simulink model "EXAMPLE"  (R2018b)
settings: Solver=ode4  StartTime=0.0  StopTime=1.8  FixedStep=50e-6  RelTol=1e-3
libraries: simulink x5, powerlib_meascontrol x5, dsparch4 x4
settings Model: Creator=Пользователь  LastModifiedBy=Пользователь

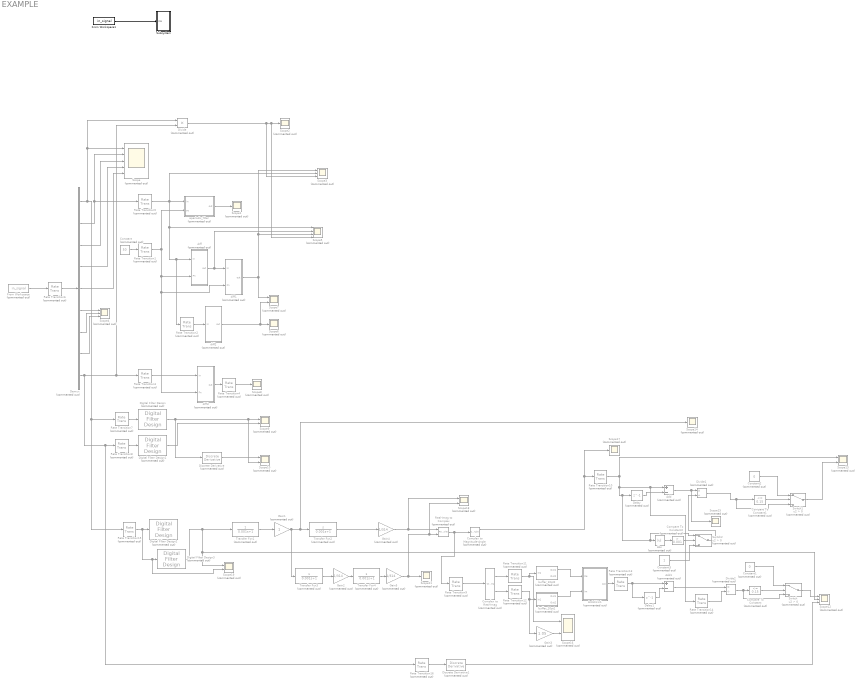
== system EXAMPLE ==
  Abs : Abs  Commented=on
  Add : Sum  Commented=on  Inputs=+-
  Add1 : Sum  Commented=on  Inputs=+-
  Antishkin1 : MATLAB Function  Commented=on  TreatAsAtomicUnit=on
  Compare To Constant : simulink/Logic and Bit Operations/Compare To Constant  Commented=on  relop=<=  const=0.15  OutDataTypeStr=boolean
  Compare To Constant1 : simulink/Logic and Bit Operations/Compare To Constant  Commented=on  relop=<=  const=0.15  OutDataTypeStr=boolean
  Compare To Constant2 : simulink/Logic and Bit Operations/Compare To Constant  Commented=on  relop=>  const=0.001  OutDataTypeStr=boolean
  Complex to Magnitude-Angle : ComplexToMagnitudeAngle  Commented=on
  Complex to Real-Imag : ComplexToRealImag  Commented=on
  Constant : Constant  Commented=on  Value=50
  Constant1 : Constant  Commented=on  Value=0
  Constant2 : Constant  Commented=on  Value=0
  Constant3 : Constant  Commented=on
  Delay : Delay  Commented=on  DelayLength=1
  Delay1 : Delay  Commented=on  DelayLength=1
  Demux : Demux  Commented=on  Outputs=9
  Digital Filter Design{,1..3} (4 alike) : dsparch4/Digital Filter Design  Commented=on  mwdsp_browser_bugfix_var=off
  Discrete Derivative : simulink/Discrete/Discrete Derivative  Commented=on  gainval=1.0  ICPrevScaledInput=0.0  OutMin=[]  OutMax=[]  OutDataType=fixdt(1, 16)  OutScaling=2^-10  DoSatur=off
  Discrete Derivative1 : simulink/Discrete/Discrete Derivative  Commented=on  gainval=1.0  ICPrevScaledInput=0.0  OutMin=[]  OutMax=[]  OutDataType=fixdt(1, 16)  OutScaling=2^-10  DoSatur=off
  Divide : Product  Commented=on  Inputs=**
  Divide1 : Product  Commented=on  Inputs=*/
  Divide2 : Product  Commented=on  Inputs=*/
  From Workspace : FromWorkspace  Commented=on  VariableName=in_signal  OutDataTypeStr=double  SampleTime=1/10000  OutputAfterFinalValue=Setting to zero
  From Workspace1 : FromWorkspace  VariableName=in_signal  OutDataTypeStr=double  SampleTime=1/10000  OutputAfterFinalValue=Setting to zero
  Gain1 : Gain  Commented=on
  Gain2 : Gain  Commented=on  Gain=1/314
  Gain3 : Gain  Commented=on  Gain=1.05
  Gain4 : Gain  Commented=on  Gain=1/314
  Gain5 : Gain  Commented=on  Gain=1/314
  Rate Transition{1..5,7..16} (15 alike) : RateTransition  Commented=on  OutPortSampleTime=1/4000
  Rate Transition6 : RateTransition  Commented=on  OutPortSampleTime=1/20000
  Real-Imag to Complex : RealImagToComplex  Commented=on
  Scope : Scope  Commented=on  NumInputPorts=5
  Scope{1..2,6,8,11,14..15,17} (8 alike) : Scope  Commented=on
  Scope{7,9..10,13,16,18..19} (7 alike) : Scope  Commented=on  NumInputPorts=2
  Scope12 : Scope  Commented=on  NumInputPorts=3
  Scope3 : Scope  Commented=on  NumInputPorts=3
  Scope4 : Scope  Commented=on  NumInputPorts=3
  Scope5 : Scope  Commented=on  NumInputPorts=4
  Subsystem : Subsystem
  Switch : Switch  Commented=on  Criteria=u2 > Threshold
  Switch1 : Switch  Commented=on  Criteria=u2 > Threshold
  Switch2 : Switch  Commented=on  Criteria=u2 > Threshold
  Transfer Fcn1 : TransferFcn  Commented=on  Numerator=1  Denominator=[0.001 1]
  Transfer Fcn2 : TransferFcn  Commented=on  Numerator=[1 0]  Denominator=[0.001 1]
  Transfer Fcn3 : TransferFcn  Commented=on  Numerator=[1 0]  Denominator=[0.001 1]
  Transfer Fcn4 : TransferFcn  Commented=on  Numerator=[1 0]  Denominator=[0.001 1]
  aperiodic_filter : Subsystem  Commented=on
  buffer_10pt1 : Subsystem  Commented=on
  buffer_10pt2 : Subsystem  Commented=on
  diff : Subsystem  Commented=on
  diff1 : Subsystem  Commented=on
  diff2 : Subsystem  Commented=on
  diff3 : Subsystem  Commented=on
  wires:
  Demux/2 -> Rate Transition5/1, Scope/2
  Demux/3 -> Scope/3
  Demux/4 -> Scope/4
  Demux/5 -> Scope/5
  aperiodic_filter/1(out) -> Scope1/1
  Constant/1 -> Rate Transition1/1
  Rate Transition5/1 -> Rate Transition2/1, diff/1(in), Scope5/1, Scope3/2, aperiodic_filter/1(in)
  Rate Transition1/1 -> aperiodic_filter/2(Fn), diff1/2(Fn), diff3/2(Fn), diff/2(Fn)
  diff/1(out) -> Scope5/2, diff1/1(in)
  diff1/1(out) -> Scope3/1, Scope5/3, Scope7/1
  Divide/1 -> Scope3/3, Scope5/4, Scope2/1
  Demux/6 -> Scope4/1
  Demux/7 -> Scope4/2
  Demux/8 -> Scope4/3
  diff2/1(out) -> Scope7/2, Scope6/1
  Rate Transition2/1 -> diff2/1(in)
  diff3/1(out) -> Rate Transition4/1
  Rate Transition3/1 -> diff3/1(in)
  Rate Transition4/1 -> Scope8/1
  Rate Transition6/1 -> Demux/1
  From Workspace/1 -> Rate Transition6/1
  Rate Transition7/1 -> Digital Filter Design/1
  Rate Transition8/1 -> Digital Filter Design1/1
  Digital Filter Design/1 -> Discrete Derivative/1, Scope10/2, Scope9/1
  Digital Filter Design1/1 -> Scope9/2
  Discrete Derivative/1 -> Scope10/1
  Transfer Fcn1/1 -> Gain1/1
  Complex to Magnitude-Angle/1 -> Scope17/1, Rate Transition10/1
  Real-Imag to Complex/1 -> Rate Transition9/1, Complex to Magnitude-Angle/1
  Rate Transition10/1 -> Scope13/1, Rate Transition14/1, Add/1, Switch2/1, Abs/1, Delay/1
  Transfer Fcn3/1 -> Gain2/1
  Complex to Real-Imag/1 -> Rate Transition11/1
  Complex to Real-Imag/2 -> Rate Transition12/1
  buffer_10pt2/1(Out1) -> Antishkin1/1(Re)
  buffer_10pt1/1(Out1) -> Antishkin1/2(Im)
  Gain1/1 -> Transfer Fcn3/1, Transfer Fcn2/1, Scope14/1
  Gain3/1 -> Scope16/2
  Demux/1 -> Rate Transition15/1, Rate Transition7/1, Divide/1, Scope/1
  Rate Transition9/1 -> Complex to Real-Imag/1
  Delay/1 -> Add/2
  Add/1 -> Scope15/1, Divide1/1
  Antishkin1/1(out) -> Rate Transition13/1
  Divide2/1 -> Switch/3, Compare To Constant/1
  Rate Transition11/1 -> Scope16/1, buffer_10pt2/1(In1)
  Rate Transition12/1 -> Gain3/1, buffer_10pt1/1(In1)
  Add1/1 -> Divide2/1
  Rate Transition14/1 -> Divide2/2
  Demux/9 -> Rate Transition16/1, Rate Transition8/1, Divide/2, Rate Transition3/1
  Compare To Constant/1 -> Switch/2
  Constant1/1 -> Switch/1
  Switch/1 -> Scope12/1
  Constant2/1 -> Switch1/1
  Compare To Constant1/1 -> Switch1/2
  Divide1/1 -> Switch1/3, Compare To Constant1/1
  Switch1/1 -> Scope13/2
  Rate Transition13/1 -> Delay1/1, Add1/1
  Delay1/1 -> Add1/2
  Gain5/1 -> Scope11/1, Scope18/2, Real-Imag to Complex/2
  Digital Filter Design3/1 -> Scope19/1, Scope12/2, Transfer Fcn1/1
  Rate Transition15/1 -> Scope19/2, Digital Filter Design3/1, Digital Filter Design2/1
  Transfer Fcn2/1 -> Gain4/1
  Gain4/1 -> Scope18/1, Real-Imag to Complex/1
  Gain2/1 -> Transfer Fcn4/1
  Transfer Fcn4/1 -> Gain5/1
  Discrete Derivative1/1 -> Scope12/3
  Rate Transition16/1 -> Discrete Derivative1/1
  Compare To Constant2/1 -> Switch2/2
  Switch2/1 -> Divide1/2
  Abs/1 -> Compare To Constant2/1
  Constant3/1 -> Switch2/3
  From Workspace1/1 -> Subsystem/1(In1)

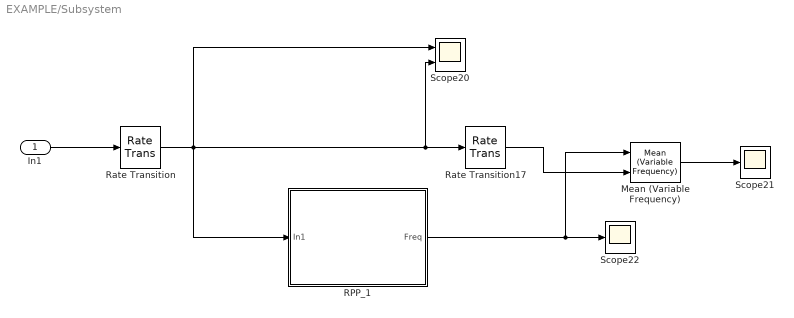
== system EXAMPLE/Subsystem ==
  In1 : Inport
  Mean (Variable Frequency) : powerlib_meascontrol/Measurements/Mean (Variable Frequency)  Finit=50  Fmin=45  Vinit=0  Ts=1/4000
      settings: SourceProductName=Simscape Power Systems  SourceProductBaseCode=PS
  RPP_1 : Subsystem
  Rate Transition : RateTransition  Integrity=off  OutPortSampleTime=1/4000
  Rate Transition17 : RateTransition  Integrity=off  OutPortSampleTime=1/4000
  Scope20 : Scope  NumInputPorts=2
  Scope21 : Scope
  Scope22 : Scope
  wires:
  Mean (Variable Frequency)/1 -> Scope21/1
  Rate Transition17/1 -> Mean (Variable Frequency)/2
  Rate Transition/1 -> RPP_1/1(In1), Rate Transition17/1, Scope20/2, Scope20/1
  RPP_1/1(Freq) -> Scope22/1, Mean (Variable Frequency)/1
  In1/1 -> Rate Transition/1

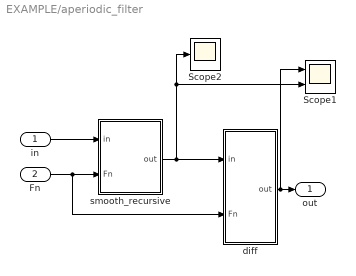
== system EXAMPLE/aperiodic_filter ==
  in : Inport
  Fn : Inport  Port=2
  Scope1 : Scope  NumInputPorts=2
  Scope2 : Scope
  diff : Subsystem
  smooth_recursive : Subsystem
  out : Outport
  wires:
  diff/1(out) -> out/1, Scope1/1
  smooth_recursive/1(out) -> diff/1(in), Scope1/2, Scope2/1
  in/1 -> smooth_recursive/1(in)
  Fn/1 -> smooth_recursive/2(Fn), diff/2(Fn)

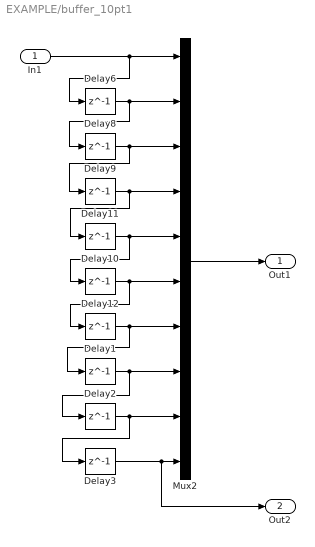
== system EXAMPLE/buffer_10pt1 ==
  In1 : Inport
  Delay{1..3,6,8..12} (9 alike) : Delay  DelayLength=1  InitialCondition=0
  Mux2 : Mux  Inputs=10
  Out1 : Outport
  Out2 : Outport  Port=2
  wires:
  Delay10/1 -> Delay12/1, Mux2/6
  Delay6/1 -> Delay8/1, Mux2/2
  Delay9/1 -> Delay11/1, Mux2/4
  Delay11/1 -> Delay10/1, Mux2/5
  Delay8/1 -> Delay9/1, Mux2/3
  Mux2/1 -> Out1/1
  Delay12/1 -> Mux2/7, Delay1/1
  Delay1/1 -> Delay2/1, Mux2/8
  Delay2/1 -> Mux2/9, Delay3/1
  Delay3/1 -> Out2/1, Mux2/10
  In1/1 -> Delay6/1, Mux2/1

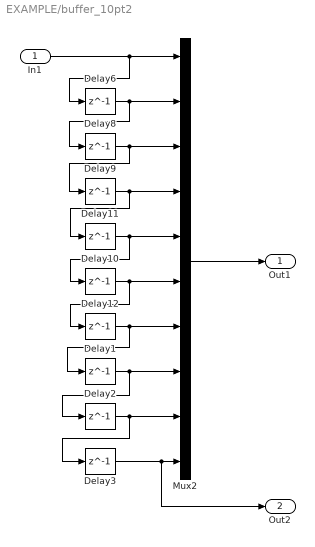
== system EXAMPLE/buffer_10pt2 ==
  In1 : Inport
  Delay{1..3,6,8..12} (9 alike) : Delay  DelayLength=1  InitialCondition=0
  Mux2 : Mux  Inputs=10
  Out1 : Outport
  Out2 : Outport  Port=2
  wires:
  In1/1 -> Mux2/1, Delay6/1
  Delay3/1 -> Mux2/10, Out2/1
  Delay2/1 -> Delay3/1, Mux2/9
  Delay1/1 -> Mux2/8, Delay2/1
  Delay12/1 -> Delay1/1, Mux2/7
  Mux2/1 -> Out1/1
  Delay8/1 -> Mux2/3, Delay9/1
  Delay11/1 -> Mux2/5, Delay10/1
  Delay9/1 -> Mux2/4, Delay11/1
  Delay6/1 -> Mux2/2, Delay8/1
  Delay10/1 -> Mux2/6, Delay12/1

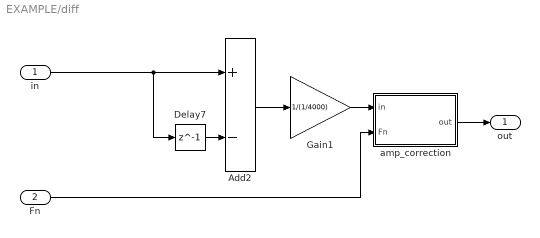
== system EXAMPLE/diff ==
  in : Inport
  Fn : Inport  Port=2
  Add2 : Sum  Inputs=+-
  Delay7 : Delay  DelayLength=1  InitialCondition=0
  Gain1 : Gain  Gain=1/(1/4000)
  amp_correction : MATLAB Function  TreatAsAtomicUnit=on
  out : Outport
  wires:
  Fn/1 -> amp_correction/2(Fn)
  in/1 -> Add2/1, Delay7/1
  Add2/1 -> Gain1/1
  Delay7/1 -> Add2/2
  Gain1/1 -> amp_correction/1(in)
  amp_correction/1(out) -> out/1

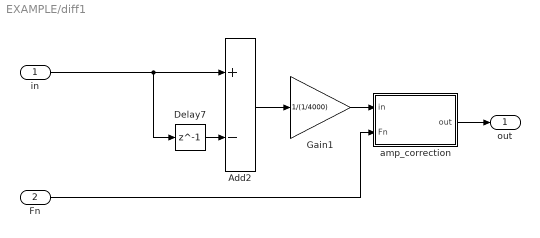
== system EXAMPLE/diff1 ==
  in : Inport
  Fn : Inport  Port=2
  Add2 : Sum  Inputs=+-
  Delay7 : Delay  DelayLength=1  InitialCondition=0
  Gain1 : Gain  Gain=1/(1/4000)
  amp_correction : MATLAB Function  TreatAsAtomicUnit=on
  out : Outport
  wires:
  amp_correction/1(out) -> out/1
  Gain1/1 -> amp_correction/1(in)
  Delay7/1 -> Add2/2
  Add2/1 -> Gain1/1
  in/1 -> Delay7/1, Add2/1
  Fn/1 -> amp_correction/2(Fn)

== system EXAMPLE/diff2 ==
  in : Inport
  Delay1 : Delay  DelayLength=1  InitialCondition=0
  Delay7 : Delay  DelayLength=1  InitialCondition=0
  Mux : Mux  Inputs=3
  amp_correction : MATLAB Function  TreatAsAtomicUnit=on
  out : Outport
  wires:
  amp_correction/1(out) -> out/1
  Mux/1 -> amp_correction/1(in)
  Delay7/1 -> Delay1/1, Mux/2
  in/1 -> Mux/1, Delay7/1
  Delay1/1 -> Mux/3

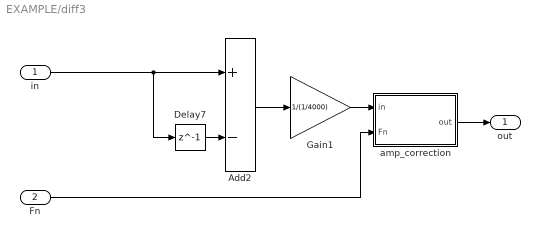
== system EXAMPLE/diff3 ==
  in : Inport
  Fn : Inport  Port=2
  Add2 : Sum  Inputs=+-
  Delay7 : Delay  DelayLength=1  InitialCondition=0
  Gain1 : Gain  Gain=1/(1/4000)
  amp_correction : MATLAB Function  TreatAsAtomicUnit=on
  out : Outport
  wires:
  amp_correction/1(out) -> out/1
  Gain1/1 -> amp_correction/1(in)
  Delay7/1 -> Add2/2
  Add2/1 -> Gain1/1
  in/1 -> Delay7/1, Add2/1
  Fn/1 -> amp_correction/2(Fn)

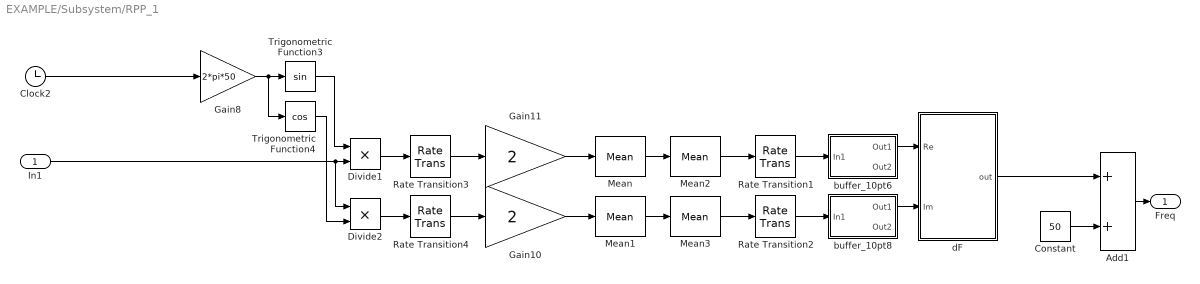
== system EXAMPLE/Subsystem/RPP_1 ==
  In1 : Inport
  Add1 : Sum
  Clock2 : Clock
  Constant : Constant  Value=50
  Divide1 : Product  Inputs=**
  Divide2 : Product  Inputs=**
  Gain10 : Gain  Gain=2
  Gain11 : Gain  Gain=2
  Gain8 : Gain  Gain=2*pi*50
  Mean : powerlib_meascontrol/Measurements/Mean  Freq=50  Vinit=0  Ts=0
  Mean1 : powerlib_meascontrol/Measurements/Mean  Freq=50  Vinit=0  Ts=0
  Mean2 : powerlib_meascontrol/Measurements/Mean  Freq=100  Vinit=0  Ts=0
  Mean3 : powerlib_meascontrol/Measurements/Mean  Freq=100  Vinit=0  Ts=0
  Rate Transition{1..4} (4 alike) : RateTransition  OutPortSampleTime=1/4000
  Trigonometric Function3 : Trigonometry
  Trigonometric Function4 : Trigonometry  Operator=cos
  buffer_10pt6 : Subsystem
  buffer_10pt8 : Subsystem
  dF : MATLAB Function  TreatAsAtomicUnit=on
  Freq : Outport
  wires:
  Mean3/1 -> Rate Transition2/1
  Rate Transition3/1 -> Gain11/1
  Divide1/1 -> Rate Transition3/1
  Clock2/1 -> Gain8/1
  Rate Transition4/1 -> Gain10/1
  buffer_10pt8/1(Out1) -> dF/2(Im)
  buffer_10pt6/1(Out1) -> dF/1(Re)
  Divide2/1 -> Rate Transition4/1
  Mean2/1 -> Rate Transition1/1
  Gain8/1 -> Trigonometric Function4/1, Trigonometric Function3/1
  Trigonometric Function3/1 -> Divide1/1
  Trigonometric Function4/1 -> Divide2/2
  dF/1(out) -> Add1/1
  Add1/1 -> Freq/1
  Constant/1 -> Add1/2
  In1/1 -> Divide2/1, Divide1/2
  Gain10/1 -> Mean1/1
  Gain11/1 -> Mean/1
  Mean/1 -> Mean2/1
  Mean1/1 -> Mean3/1
  Rate Transition1/1 -> buffer_10pt6/1(In1)
  Rate Transition2/1 -> buffer_10pt8/1(In1)

== system EXAMPLE/aperiodic_filter/diff ==
  in : Inport
  Fn : Inport  Port=2
  Add2 : Sum  Inputs=+-
  Delay7 : Delay  DelayLength=1  InitialCondition=0
  Gain1 : Gain  Gain=1/(1/4000)
  amp_correction : MATLAB Function  TreatAsAtomicUnit=on
  out : Outport
  wires:
  Fn/1 -> amp_correction/2(Fn)
  amp_correction/1(out) -> out/1
  in/1 -> Add2/1, Delay7/1
  Add2/1 -> Gain1/1
  Delay7/1 -> Add2/2
  Gain1/1 -> amp_correction/1(in)

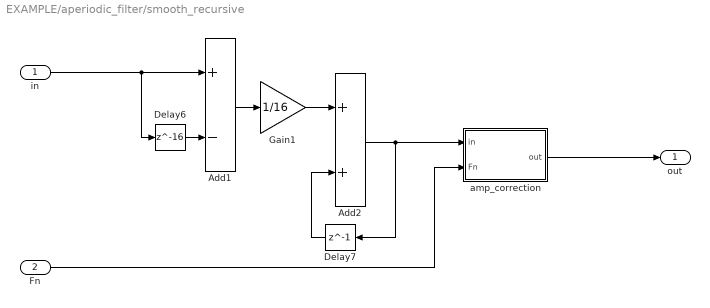
== system EXAMPLE/aperiodic_filter/smooth_recursive ==
  in : Inport
  Fn : Inport  Port=2
  Add1 : Sum  Inputs=+-
  Add2 : Sum
  Delay6 : Delay  DelayLength=16  InitialCondition=0
  Delay7 : Delay  DelayLength=1  InitialCondition=0
  Gain1 : Gain  Gain=1/16
  amp_correction : MATLAB Function  TreatAsAtomicUnit=on
  out : Outport
  wires:
  Fn/1 -> amp_correction/2(Fn)
  amp_correction/1(out) -> out/1
  Delay7/1 -> Add2/2
  in/1 -> Add1/1, Delay6/1
  Add1/1 -> Gain1/1
  Delay6/1 -> Add1/2
  Add2/1 -> Delay7/1, amp_correction/1(in)
  Gain1/1 -> Add2/1

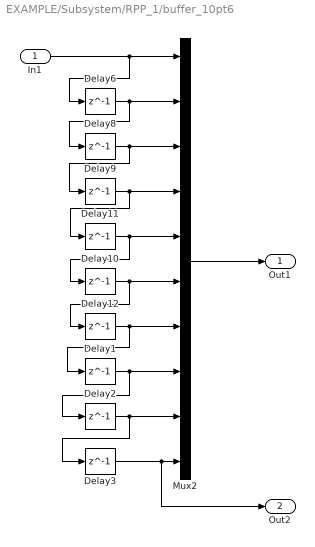
== system EXAMPLE/Subsystem/RPP_1/buffer_10pt6 ==
  In1 : Inport
  Delay{1..3,6,8..12} (9 alike) : Delay  DelayLength=1  InitialCondition=0
  Mux2 : Mux  Inputs=10
  Out1 : Outport
  Out2 : Outport  Port=2
  wires:
  In1/1 -> Mux2/1, Delay6/1
  Delay3/1 -> Mux2/10, Out2/1
  Delay2/1 -> Delay3/1, Mux2/9
  Delay1/1 -> Mux2/8, Delay2/1
  Delay12/1 -> Delay1/1, Mux2/7
  Mux2/1 -> Out1/1
  Delay8/1 -> Mux2/3, Delay9/1
  Delay11/1 -> Mux2/5, Delay10/1
  Delay9/1 -> Mux2/4, Delay11/1
  Delay6/1 -> Mux2/2, Delay8/1
  Delay10/1 -> Mux2/6, Delay12/1

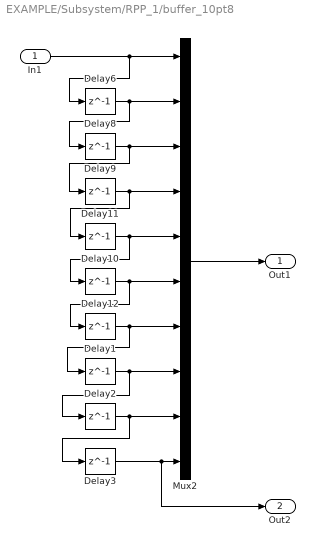
== system EXAMPLE/Subsystem/RPP_1/buffer_10pt8 ==
  In1 : Inport
  Delay{1..3,6,8..12} (9 alike) : Delay  DelayLength=1  InitialCondition=0
  Mux2 : Mux  Inputs=10
  Out1 : Outport
  Out2 : Outport  Port=2
  wires:
  Delay10/1 -> Delay12/1, Mux2/6
  Delay6/1 -> Delay8/1, Mux2/2
  Delay9/1 -> Delay11/1, Mux2/4
  Delay11/1 -> Delay10/1, Mux2/5
  Delay8/1 -> Delay9/1, Mux2/3
  Mux2/1 -> Out1/1
  Delay12/1 -> Mux2/7, Delay1/1
  Delay1/1 -> Delay2/1, Mux2/8
  Delay2/1 -> Mux2/9, Delay3/1
  Delay3/1 -> Out2/1, Mux2/10
  In1/1 -> Delay6/1, Mux2/1

== matlab function EXAMPLE/diff/amp_correction ==
  data: in input; out output; Fn input
function out   = fcn(in , Fn)

% Исходные данные:
Fs       = 4000;

ReDRV = ( 1 - cos(-2*pi*1*Fn/Fs) )/(1/Fs);
ImDRV = ( 0 - sin(-2*pi*1*Fn/Fs) )/(1/Fs);

%Считаем ослабленную амплитуду входного единичного сигнала:
KmDRV = sqrt( ReDRV^2 + ImDRV^2 );

%Считаем коэффициент ослабления спектра входного единичного сигнала:
out      = in/KmDRV;

end

== matlab function EXAMPLE/diff1/amp_correction ==
  data: in input; out output; Fn input
function out   = fcn(in , Fn)

% Исходные данные:
Fs       = 4000;

ReDRV = ( 1 - cos(-2*pi*1*Fn/Fs) )/(1/Fs);
ImDRV = ( 0 - sin(-2*pi*1*Fn/Fs) )/(1/Fs);

%Считаем ослабленную амплитуду входного единичного сигнала:
KmDRV = sqrt( ReDRV^2 + ImDRV^2 );

%Считаем коэффициент ослабления спектра входного единичного сигнала:
out      = in/KmDRV;

end

== matlab function EXAMPLE/diff2/amp_correction ==
  data: in input; out output
function out   = fcn(in)

% Исходные данные:
Fs       = 4000;

Km  = - 2 * ( cos(2*pi*50/4000) - 1);

out = 0;

%if( abs(in(1)) > 0.001 && abs(in(2)) > 0.001 && abs(in(3)) > 0.001 )
out = ( in(1) + in(3) - 2*in(2) ) / Km; 
%end

end

== matlab function EXAMPLE/diff3/amp_correction ==
  data: in input; out output; Fn input
function out   = fcn(in , Fn)

% Исходные данные:
Fs       = 4000;

ReDRV = ( 1 - cos(-2*pi*1*Fn/Fs) )/(1/Fs);
ImDRV = ( 0 - sin(-2*pi*1*Fn/Fs) )/(1/Fs);

%Считаем ослабленную амплитуду входного единичного сигнала:
KmDRV = sqrt( ReDRV^2 + ImDRV^2 );

%Считаем коэффициент ослабления спектра входного единичного сигнала:
out      = in/KmDRV;

end

== matlab function EXAMPLE/Subsystem/RPP_1/dF ==
  data: Re input; out output; Im input
function out   = fcn(Re , Im)

V1 = Re(1) + 1i * Im(1);
V2 = Re(2) - 1i * Im(2);

dVmlpx = V1 * V2;

out  = 50 * angle(dVmlpx) * 80 / 1 / 2 / pi;

end

== matlab function EXAMPLE/aperiodic_filter/smooth_recursive/amp_correction ==
  data: in input; out output; Fn input
function out   = fcn(in , Fn)

% Исходные данные:
Fs       = 4000;

%Рассчитываем АЧХ сглаживающего КИХ - фильтра:
ReSMOOTH = 0;
ImSMOOTH = 0;

for n = 1:1:16
ReSMOOTH = ReSMOOTH + cos(-2*pi*(n-1)*Fn/Fs) ;
ImSMOOTH = ImSMOOTH + sin(-2*pi*(n-1)*Fn/Fs) ;
end

%Считаем ослабленную амплитуду входного единичного сигнала:
KmSMOOTH = sqrt( ReSMOOTH^2 + ImSMOOTH^2 );

%Считаем коэффициент ослабления спектра входного единичного сигнала:
out      = in*16/KmSMOOTH;

end

== matlab function EXAMPLE/aperiodic_filter/diff/amp_correction ==
  data: in input; out output; Fn input
function out   = fcn(in , Fn)

% Исходные данные:
Fs       = 4000;

ReDRV = ( 1 - cos(-2*pi*1*Fn/Fs) )/(1/Fs);
ImDRV = ( 0 - sin(-2*pi*1*Fn/Fs) )/(1/Fs);

%Считаем ослабленную амплитуду входного единичного сигнала:
KmDRV = sqrt( ReDRV^2 + ImDRV^2 );

%Считаем коэффициент ослабления спектра входного единичного сигнала:
out      = in/KmDRV;

end

== matlab function EXAMPLE/Antishkin1 ==
  data: Re input; out output; Im input
function out   = fcn(Re, Im)


out = sqrt( abs( Re(1)^2 + Im(1)^2 + Re(2)^2 + Im(2)^2 - 2*( Re(1)*Re(2) + Im(1)*Im(2) ) ) );

end
